simulink model "FirstOrderNomoto"  (R2023a)
settings: Solver=VariableStepAuto  StartTime=0.0  StopTime=10  RelTol=1e-3
settings Model: Creator=ruben  LastModifiedBy=ruben

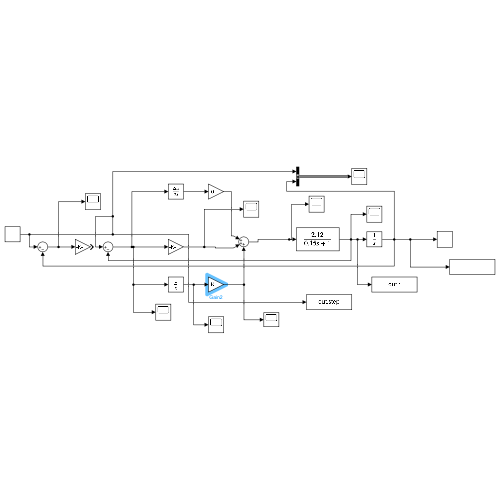
[thumbnail: Simulink's stored preview of the top-level diagram]
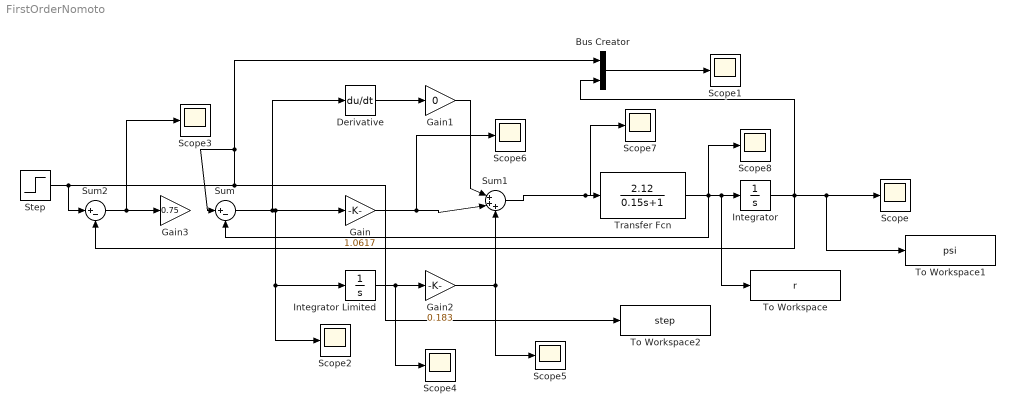
== system FirstOrderNomoto ==
  Bus Creator : BusCreator  Inputs=2
  Derivative : Derivative
  Gain : Gain  Gain=1.0617
  Gain1 : Gain  Gain=0
  Gain2 : Gain  Gain=0.183
  Gain3 : Gain  Gain=0.75
  Integrator : Integrator
  Integrator Limited : Integrator  UpperSaturationLimit=1  LowerSaturationLimit=0
  Scope{,1..8} (9 alike) : Scope
  Step : Step  After=10  SampleTime=0
  Sum : Sum  Inputs=|+-
  Sum1 : Sum  Inputs=|+++
  Sum2 : Sum  Inputs=|+-
  To Workspace : ToWorkspace  VariableName=r  SaveFormat=Timeseries  SampleTime=-1
  To Workspace1 : ToWorkspace  VariableName=psi  SaveFormat=Timeseries  SampleTime=-1
  To Workspace2 : ToWorkspace  VariableName=step  SaveFormat=Timeseries  SampleTime=-1
  Transfer Fcn : TransferFcn  Numerator=[2.12]  Denominator=[0.15 1]
  wires:
  Derivative/1 -> Gain1/1
  Gain2/1 -> Scope5/1, Sum1/3
  Gain1/1 -> Sum1/1
  Integrator Limited/1 -> Scope4/1, Gain2/1
  Sum2/1 -> Gain3/1, Scope3/1
  Integrator/1 -> Sum2/2, Bus Creator/2, To Workspace1/1, Scope/1
  Sum/1 -> Derivative/1, Scope2/1, Integrator Limited/1, Gain/1
  Gain/1 -> Sum1/2, Scope6/1
  Sum1/1 -> Scope7/1, Transfer Fcn/1
  Bus Creator/1 -> Scope1/1
  Transfer Fcn/1 -> Scope8/1, Sum/2, To Workspace/1, Integrator/1
  Step/1 -> To Workspace2/1, Sum/1, Bus Creator/1, Sum2/1
